simulink model "IEEE9Buses"  (R2024b)
settings: Solver=FixedStepAuto  StartTime=0  StopTime=5  FixedStep=1e-6  RelTol=1e-3
values from neighbouring files (symbols this model uses):
  SG_D_1_D = 0.01056    [SG9_parameters.m]
  SG_D_1_EnableSaturation = 0    [SG9_parameters.m]
  SG_D_1_f0 = 60    [SG9_parameters.m]
  SG_D_1_H = 7.5    [SG9_parameters.m]
  SG_D_1_K_A = 20    [SG9_parameters.m]
  SG_D_1_K_E = 1.000000e+1    (= 10)    [SG9_parameters.m]
  SG_D_1_K_F = 2.363    [SG9_parameters.m]
  SG_D_1_K_s = 5    [SG9_parameters.m]
  SG_D_1_R_a = 0.001088    [SG9_parameters.m]
  SG_D_1_S_A = 1    [SG9_parameters.m]
  SG_D_1_S_B = 0.103    [SG9_parameters.m]
  SG_D_1_S_N = 10.659857    [SG9_parameters.m]
  SG_D_1_SpeedPara = 200    [SG9_parameters.m]
  SG_D_1_T_0 = 0.720173    [SG9_parameters.m]
  SG_D_1_T_1 = 0.3    [SG9_parameters.m]
  SG_D_1_T_2 = 0.05    [SG9_parameters.m]
  SG_D_1_T_3 = 0.02    [SG9_parameters.m]
  SG_D_1_T_4 = 0.005    [SG9_parameters.m]
  SG_D_1_T_A = 0.02    [SG9_parameters.m]
  SG_D_1_T_dd = 8.000000e+0    (= 8)    [SG9_parameters.m]
  SG_D_1_T_ddd = 0.04    [SG9_parameters.m]
  SG_D_1_T_E = 0.314    [SG9_parameters.m]
  SG_D_1_T_F = 0.35    [SG9_parameters.m]
  SG_D_1_T_qd = 0.8    [SG9_parameters.m]
  SG_D_1_T_qdd = 0.02    [SG9_parameters.m]
  SG_D_1_T_speed = 0.1    [SG9_parameters.m]
  SG_D_1_T_w = 0.5    [SG9_parameters.m]
  SG_D_1_V_ref = 1.990276    [SG9_parameters.m]
  SG_D_1_w_ref = 376.991118    [SG9_parameters.m]
  SG_D_1_x_d = 1.9    [SG9_parameters.m]
  SG_D_1_x_dd = 0.302    [SG9_parameters.m]
  SG_D_1_x_ddd = 0.204    [SG9_parameters.m]
  SG_D_1_x_l = 0.05    [SG9_parameters.m]
  SG_D_1_x_q = 1.3    [SG9_parameters.m]
  SG_D_1_x_qd = 0.5    [SG9_parameters.m]
  SG_D_1_x_qdd = 0.3    [SG9_parameters.m]
  SG_D_2_D = 0.01056    [SG9_parameters.m]
  SG_D_2_EnableSaturation = 0    [SG9_parameters.m]
  SG_D_2_f0 = 60    [SG9_parameters.m]
  SG_D_2_H = 7.5    [SG9_parameters.m]
  SG_D_2_K_A = 20    [SG9_parameters.m]
  SG_D_2_K_E = 1.000000e+1    (= 10)    [SG9_parameters.m]
  SG_D_2_K_F = 2.363    [SG9_parameters.m]
  SG_D_2_K_s = 0.5    [SG9_parameters.m]
  SG_D_2_R_a = 0.001088    [SG9_parameters.m]
  SG_D_2_S_A = 1    [SG9_parameters.m]
  SG_D_2_S_B = 0.103    [SG9_parameters.m]
  SG_D_2_S_N = 10.659857    [SG9_parameters.m]
  SG_D_2_SpeedPara = 200    [SG9_parameters.m]
  SG_D_2_T_0 = 1.632913    [SG9_parameters.m]
  SG_D_2_T_1 = 0.2    [SG9_parameters.m]
  SG_D_2_T_2 = 0.05    [SG9_parameters.m]
  SG_D_2_T_3 = 0.02    [SG9_parameters.m]
  SG_D_2_T_4 = 0.005    [SG9_parameters.m]
  SG_D_2_T_A = 0.02    [SG9_parameters.m]
  SG_D_2_T_dd = 8.000000e+0    (= 8)    [SG9_parameters.m]
  SG_D_2_T_ddd = 0.04    [SG9_parameters.m]
  SG_D_2_T_E = 0.314    [SG9_parameters.m]
  SG_D_2_T_F = 0.35    [SG9_parameters.m]
  SG_D_2_T_qd = 0.8    [SG9_parameters.m]
  SG_D_2_T_qdd = 0.02    [SG9_parameters.m]
  SG_D_2_T_speed = 0.1    [SG9_parameters.m]
  SG_D_2_T_w = 0.5    [SG9_parameters.m]
  SG_D_2_V_ref = 2.662631    [SG9_parameters.m]
  SG_D_2_w_ref = 376.991118    [SG9_parameters.m]
  SG_D_2_x_d = 1.9    [SG9_parameters.m]
  SG_D_2_x_dd = 0.302    [SG9_parameters.m]
  SG_D_2_x_ddd = 0.204    [SG9_parameters.m]
  SG_D_2_x_l = 0.05    [SG9_parameters.m]
  SG_D_2_x_q = 1.3    [SG9_parameters.m]
  SG_D_2_x_qd = 0.5    [SG9_parameters.m]
  SG_D_2_x_qdd = 0.3    [SG9_parameters.m]
  SG_D_3_D = 0.01056    [SG9_parameters.m]
  SG_D_3_EnableSaturation = 0    [SG9_parameters.m]
  SG_D_3_f0 = 60    [SG9_parameters.m]
  SG_D_3_H = 7.5    [SG9_parameters.m]
  SG_D_3_K_A = 20    [SG9_parameters.m]
  SG_D_3_K_E = 1.000000e+1    (= 10)    [SG9_parameters.m]
  SG_D_3_K_F = 2.363    [SG9_parameters.m]
  SG_D_3_K_s = 0.5    [SG9_parameters.m]
  SG_D_3_R_a = 0.001088    [SG9_parameters.m]
  SG_D_3_S_A = 1    [SG9_parameters.m]
  SG_D_3_S_B = 0.103    [SG9_parameters.m]
  SG_D_3_S_N = 10.659857    [SG9_parameters.m]
  SG_D_3_SpeedPara = 200    [SG9_parameters.m]
  SG_D_3_T_0 = 0.850788    [SG9_parameters.m]
  SG_D_3_T_1 = 0.2    [SG9_parameters.m]
  SG_D_3_T_2 = 0.05    [SG9_parameters.m]
  SG_D_3_T_3 = 0.02    [SG9_parameters.m]
  SG_D_3_T_4 = 0.005    [SG9_parameters.m]
  SG_D_3_T_A = 0.02    [SG9_parameters.m]
  SG_D_3_T_dd = 8.000000e+0    (= 8)    [SG9_parameters.m]
  SG_D_3_T_ddd = 0.04    [SG9_parameters.m]
  SG_D_3_T_E = 0.314    [SG9_parameters.m]
  SG_D_3_T_F = 0.35    [SG9_parameters.m]
  SG_D_3_T_qd = 0.8    [SG9_parameters.m]
  SG_D_3_T_qdd = 0.02    [SG9_parameters.m]
  SG_D_3_T_speed = 0.1    [SG9_parameters.m]
  SG_D_3_T_w = 0.5    [SG9_parameters.m]
  SG_D_3_V_ref = 1.915682    [SG9_parameters.m]
  SG_D_3_w_ref = 376.991118    [SG9_parameters.m]
  SG_D_3_x_d = 1.9    [SG9_parameters.m]
  SG_D_3_x_dd = 0.302    [SG9_parameters.m]
  SG_D_3_x_ddd = 0.204    [SG9_parameters.m]
  SG_D_3_x_l = 0.05    [SG9_parameters.m]
  SG_D_3_x_q = 1.3    [SG9_parameters.m]
  SG_D_3_x_qd = 0.5    [SG9_parameters.m]
  SG_D_3_x_qdd = 0.3    [SG9_parameters.m]
(part 9 of 9)

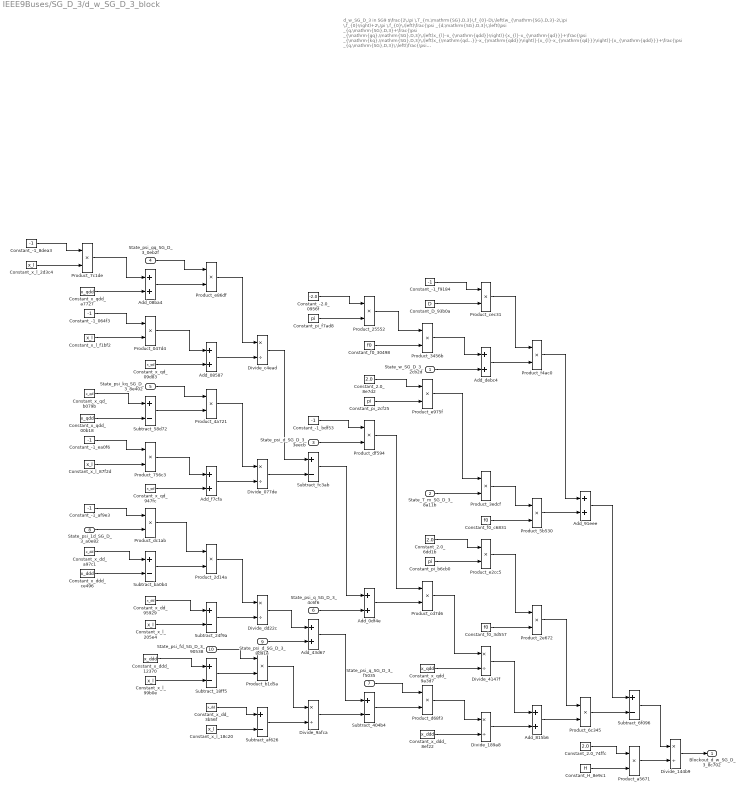
== system IEEE9Buses/SG_D_3/d_w_SG_D_3_block ==
  note: d_w_SG_D_3 in SG9
      | $\frac{2\,\pi \,T_{m,\mathrm{SG},D,3}\,f_{0}-D\,\left(w_{\mathrm{SG},D,3}-2\,\pi \,f_{0}\right)+2\,\pi \,f_{0}\,\left(\frac{\psi _{d,\mathrm{SG},D,3}\,\left(\psi _{q,\mathrm{SG},D,3}+\frac{\psi _{\mathrm{gq},\mathrm{SG},D,3}\,\left(x_{l}-x_{\mathrm{qdd}}\right)}{x_{l}-x_{\mathrm{qd}}}+\frac{\psi _{\mathrm{kq},\mathrm{SG},D,3}\,\left(x_{\mathrm{qd}}-x_{\mathrm{qdd}}\right)}{x_{l}-x_{\mathrm{qd}}}\right)}{x_{\mathrm{qdd}}}+\frac{\psi _{q,\mathrm{SG},D,3}\,\left(\frac{\psi _{\mathrm{1d},\mathrm{SG},D,3}\,\left(x_{\mathrm{dd}}-x_{\mathrm{ddd}}\right)}{x_{\mathrm{dd}}-x_{l}}-\psi _{d,\mathrm{SG},D,3}+\frac{\psi _{\mathrm{fd},\mathrm{SG},D,3}\,\left(x_{\mathrm{ddd}}-x_{l}\right)}{x_{\mathrm{dd}}-x_{l}}\right)}{x_{\mathrm{ddd}}}\right)}{2\,H}$
      | Automatically generated on 2025-09-12 21:33:31 .
  State_w_SG_D_3_2cb2d : Inport
  State_T_m_SG_D_3_8a11b : Inport  Port=2
  State_psi_d_SG_D_3_3eecb : Inport  Port=3
  State_psi_gq_SG_D_3_0eb2f : Inport  Port=4
  State_psi_kq_SG_D_3_8e402 : Inport  Port=5
  State_psi_q_SG_D_3_4c6f6 : Inport  Port=6
  State_psi_q_SG_D_3_f5035 : Inport  Port=7
  State_psi_1d_SG_D_3_a0e82 : Inport  Port=8
  State_psi_d_SG_D_3_8d91e : Inport  Port=9
  State_psi_fd_SG_D_3_90538 : Inport  Port=10
  Add_08587 : Sum
  Add_08ba4 : Sum
  Add_0df4e : Sum
  Add_43d67 : Sum
  Add_815b6 : Sum
  Add_91eee : Sum
  Add_debc4 : Sum
  Add_f7cfa : Sum
  Constant_-1_064f3 : Constant  Value=-1
  Constant_-1_8dea3 : Constant  Value=-1
  Constant_-1_af9e3 : Constant  Value=-1
  Constant_-1_bdf53 : Constant  Value=-1
  Constant_-1_ea0f6 : Constant  Value=-1
  Constant_-1_f9184 : Constant  Value=-1
  Constant_-2.0_0956f : Constant  Value=-2.0
  Constant_2.0_6dd1b : Constant  Value=2.0
  Constant_2.0_74ffc : Constant  Value=2.0
  Constant_2.0_8e7d2 : Constant  Value=2.0
  Constant_D_93b0a : Constant  Value=D
  Constant_H_8e9c1 : Constant  Value=H
  Constant_f0_30498 : Constant  Value=f0
  Constant_f0_3d557 : Constant  Value=f0
  Constant_f0_c6831 : Constant  Value=f0
  Constant_pi_2cf25 : Constant  Value=pi
  Constant_pi_b6cb0 : Constant  Value=pi
  Constant_pi_f7ad8 : Constant  Value=pi
  Constant_x_dd_3b56f : Constant  Value=x_dd
  Constant_x_dd_95929 : Constant  Value=x_dd
  Constant_x_dd_a97c1 : Constant  Value=x_dd
  Constant_x_ddd_12370 : Constant  Value=x_ddd
  Constant_x_ddd_8ef22 : Constant  Value=x_ddd
  Constant_x_ddd_ce496 : Constant  Value=x_ddd
  Constant_x_l_18c20 : Constant  Value=x_l
  Constant_x_l_205e4 : Constant  Value=x_l
  Constant_x_l_2d3c4 : Constant  Value=x_l
  Constant_x_l_87f2d : Constant  Value=x_l
  Constant_x_l_99b0e : Constant  Value=x_l
  Constant_x_l_f1bf2 : Constant  Value=x_l
  Constant_x_qd_09d83 : Constant  Value=x_qd
  Constant_x_qd_947fc : Constant  Value=x_qd
  Constant_x_qd_b079b : Constant  Value=x_qd
  Constant_x_qdd_00b18 : Constant  Value=x_qdd
  Constant_x_qdd_9a3d7 : Constant  Value=x_qdd
  Constant_x_qdd_a7727 : Constant  Value=x_qdd
  Divide_077de : Product  Inputs=*/
  Divide_144b9 : Product  Inputs=*/
  Divide_189a8 : Product  Inputs=*/
  Divide_4147f : Product  Inputs=*/
  Divide_9afca : Product  Inputs=*/
  Divide_c4ead : Product  Inputs=*/
  Divide_dd22c : Product  Inputs=*/
  Product_047d4 : Product
  Product_25552 : Product
  Product_2d14a : Product
  Product_2e672 : Product
  Product_3456b : Product
  Product_3edcf : Product
  Product_4a721 : Product
  Product_5b530 : Product
  Product_6c345 : Product
  Product_756c3 : Product
  Product_7c1de : Product
  Product_a5671 : Product
  Product_b1d5a : Product
  Product_cd7d6 : Product
  Product_cec31 : Product
  Product_d68f3 : Product
  Product_dc1ab : Product
  Product_df594 : Product
  Product_e2cc5 : Product
  Product_e86df : Product
  Product_e975f : Product
  Product_f4ac0 : Product
  Subtract_18ff5 : Sum  Inputs=+-
  Subtract_24f9a : Sum  Inputs=+-
  Subtract_404b4 : Sum  Inputs=+-
  Subtract_58d72 : Sum  Inputs=+-
  Subtract_6f096 : Sum  Inputs=+-
  Subtract_af626 : Sum  Inputs=+-
  Subtract_ba0b4 : Sum  Inputs=+-
  Subtract_fc3ab : Sum  Inputs=+-
  Blockout_d_w_SG_D_3_8c702 : Outport
  wires:
  Constant_x_qd_b079b/1 -> Subtract_58d72/1
  Subtract_ba0b4/1 -> Product_2d14a/2
  Subtract_6f096/1 -> Divide_144b9/1
  Constant_-1_8dea3/1 -> Product_7c1de/1
  Add_08ba4/1 -> Product_e86df/2
  Constant_x_qdd_00b18/1 -> Subtract_58d72/2
  Subtract_18ff5/1 -> Product_b1d5a/2
  Constant_x_l_2d3c4/1 -> Product_7c1de/2
  State_psi_d_SG_D_3_8d91e/1 -> Add_43d67/2
  Add_08587/1 -> Divide_c4ead/2
  Constant_x_dd_95929/1 -> Subtract_24f9a/1
  Constant_x_l_f1bf2/1 -> Product_047d4/2
  Constant_-1_f9184/1 -> Product_cec31/1
  Divide_9afca/1 -> Subtract_404b4/2
  Constant_x_ddd_ce496/1 -> Subtract_ba0b4/2
  Constant_x_qdd_a7727/1 -> Add_08ba4/2
  Constant_pi_2cf25/1 -> Product_e975f/2
  Product_7c1de/1 -> Add_08ba4/1
  Constant_-2.0_0956f/1 -> Product_25552/1
  Constant_-1_064f3/1 -> Product_047d4/1
  Constant_2.0_6dd1b/1 -> Product_e2cc5/1
  Product_25552/1 -> Product_3456b/1
  Constant_-1_ea0f6/1 -> Product_756c3/1
  Subtract_fc3ab/1 -> Add_0df4e/1
  Constant_x_l_87f2d/1 -> Product_756c3/2
  Constant_x_l_99b0e/1 -> Subtract_18ff5/2
  Constant_-1_af9e3/1 -> Product_dc1ab/1
  State_psi_1d_SG_D_3_a0e82/1 -> Product_dc1ab/2
  Constant_x_dd_a97c1/1 -> Subtract_ba0b4/1
  Product_dc1ab/1 -> Product_2d14a/1
  State_psi_gq_SG_D_3_0eb2f/1 -> Product_e86df/1
  Constant_x_qd_09d83/1 -> Add_08587/2
  Product_047d4/1 -> Add_08587/1
  State_psi_kq_SG_D_3_8e402/1 -> Product_4a721/1
  Subtract_58d72/1 -> Product_4a721/2
  Product_e2cc5/1 -> Product_2e672/1
  Product_3456b/1 -> Add_debc4/1
  Product_756c3/1 -> Add_f7cfa/1
  State_psi_q_SG_D_3_f5035/1 -> Product_d68f3/1
  Constant_x_qd_947fc/1 -> Add_f7cfa/2
  Constant_x_l_205e4/1 -> Subtract_24f9a/2
  Constant_x_ddd_12370/1 -> Subtract_18ff5/1
  Constant_x_l_18c20/1 -> Subtract_af626/2
  Product_e86df/1 -> Divide_c4ead/1
  Product_4a721/1 -> Divide_077de/1
  Add_f7cfa/1 -> Divide_077de/2
  Product_2d14a/1 -> Divide_dd22c/1
  Subtract_24f9a/1 -> Divide_dd22c/2
  Constant_2.0_8e7d2/1 -> Product_e975f/1
  State_psi_fd_SG_D_3_90538/1 -> Product_b1d5a/1
  Constant_x_dd_3b56f/1 -> Subtract_af626/1
  Divide_c4ead/1 -> Subtract_fc3ab/1
  Product_b1d5a/1 -> Divide_9afca/1
  Divide_077de/1 -> Subtract_fc3ab/2
  Divide_dd22c/1 -> Add_43d67/1
  Product_6c345/1 -> Subtract_6f096/2
  Subtract_af626/1 -> Divide_9afca/2
  Constant_pi_f7ad8/1 -> Product_25552/2
  Constant_pi_b6cb0/1 -> Product_e2cc5/2
  Constant_-1_bdf53/1 -> Product_df594/1
  State_psi_d_SG_D_3_3eecb/1 -> Product_df594/2
  State_psi_q_SG_D_3_4c6f6/1 -> Add_0df4e/2
  Add_43d67/1 -> Subtract_404b4/1
  Constant_f0_30498/1 -> Product_3456b/2
  Product_df594/1 -> Product_cd7d6/1
  Add_0df4e/1 -> Product_cd7d6/2
  Subtract_404b4/1 -> Product_d68f3/2
  Constant_D_93b0a/1 -> Product_cec31/2
  State_w_SG_D_3_2cb2d/1 -> Add_debc4/2
  Product_e975f/1 -> Product_3edcf/1
  State_T_m_SG_D_3_8a11b/1 -> Product_3edcf/2
  Product_cd7d6/1 -> Divide_4147f/1
  Constant_x_qdd_9a3d7/1 -> Divide_4147f/2
  Product_d68f3/1 -> Divide_189a8/1
  Constant_x_ddd_8ef22/1 -> Divide_189a8/2
  Product_cec31/1 -> Product_f4ac0/1
  Add_debc4/1 -> Product_f4ac0/2
  Product_3edcf/1 -> Product_5b530/1
  Constant_f0_c6831/1 -> Product_5b530/2
  Constant_f0_3d557/1 -> Product_2e672/2
  Divide_4147f/1 -> Add_815b6/1
  Divide_189a8/1 -> Add_815b6/2
  Product_f4ac0/1 -> Add_91eee/1
  Product_5b530/1 -> Add_91eee/2
  Product_2e672/1 -> Product_6c345/1
  Add_815b6/1 -> Product_6c345/2
  Add_91eee/1 -> Subtract_6f096/1
  Constant_2.0_74ffc/1 -> Product_a5671/1
  Constant_H_8e9c1/1 -> Product_a5671/2
  Product_a5671/1 -> Divide_144b9/2
  Divide_144b9/1 -> Blockout_d_w_SG_D_3_8c702/1

== system IEEE9Buses/SG_D_3/i_d_SG_D_3_block ==
  note: i_d_SG_D_3 in SG9
      | $\frac{\sin\left(\theta _{\mathrm{SG},D,3}\right)\,\left(\frac{\psi _{\mathrm{1d},\mathrm{SG},D,3}\,\left(x_{\mathrm{dd}}-x_{\mathrm{ddd}}\right)}{x_{\mathrm{dd}}-x_{l}}-\psi _{d,\mathrm{SG},D,3}+\frac{\psi _{\mathrm{fd},\mathrm{SG},D,3}\,\left(x_{\mathrm{ddd}}-x_{l}\right)}{x_{\mathrm{dd}}-x_{l}}\right)}{x_{\mathrm{ddd}}}-\frac{\cos\left(\theta _{\mathrm{SG},D,3}\right)\,\left(\psi _{q,\mathrm{SG},D,3}+\frac{\psi _{\mathrm{gq},\mathrm{SG},D,3}\,\left(x_{l}-x_{\mathrm{qdd}}\right)}{x_{l}-x_{\mathrm{qd}}}+\frac{\psi _{\mathrm{kq},\mathrm{SG},D,3}\,\left(x_{\mathrm{qd}}-x_{\mathrm{qdd}}\right)}{x_{l}-x_{\mathrm{qd}}}\right)}{x_{\mathrm{qdd}}}$
      | Automatically generated on 2025-09-12 21:33:53 .
  State_psi_gq_SG_D_3_f9205 : Inport
  State_psi_kq_SG_D_3_f6fb5 : Inport  Port=2
  State_psi_q_SG_D_3_097ac : Inport  Port=3
  State_theta_SG_D_3_f2e5f : Inport  Port=4
  State_psi_1d_SG_D_3_3346a : Inport  Port=5
  State_psi_d_SG_D_3_c47d7 : Inport  Port=6
  State_psi_fd_SG_D_3_3705f : Inport  Port=7
  State_theta_SG_D_3_0b124 : Inport  Port=8
  Add_2e819 : Sum
  Add_66e39 : Sum
  Add_78c11 : Sum
  Add_abcc7 : Sum
  Add_c4e16 : Sum
  Constant_-1_12cb5 : Constant  Value=-1
  Constant_-1_21ee1 : Constant  Value=-1
  Constant_-1_82b40 : Constant  Value=-1
  Constant_-1_ad0d8 : Constant  Value=-1
  Constant_-1_b0e43 : Constant  Value=-1
  Constant_x_dd_4f659 : Constant  Value=x_dd
  Constant_x_dd_899e7 : Constant  Value=x_dd
  Constant_x_dd_a714f : Constant  Value=x_dd
  Constant_x_ddd_259a3 : Constant  Value=x_ddd
  Constant_x_ddd_74b9b : Constant  Value=x_ddd
  Constant_x_ddd_a6c9b : Constant  Value=x_ddd
  Constant_x_l_212b9 : Constant  Value=x_l
  Constant_x_l_37c3f : Constant  Value=x_l
  Constant_x_l_510f9 : Constant  Value=x_l
  Constant_x_l_60d37 : Constant  Value=x_l
  Constant_x_l_90ef1 : Constant  Value=x_l
  Constant_x_l_ade82 : Constant  Value=x_l
  Constant_x_qd_06573 : Constant  Value=x_qd
  Constant_x_qd_86486 : Constant  Value=x_qd
  Constant_x_qd_d7580 : Constant  Value=x_qd
  Constant_x_qdd_3a2d2 : Constant  Value=x_qdd
  Constant_x_qdd_a541f : Constant  Value=x_qdd
  Constant_x_qdd_c4b29 : Constant  Value=x_qdd
  Divide_d5013 : Product  Inputs=*/
  Divide_d79b9 : Product  Inputs=*/
  Divide_d802b : Product  Inputs=*/
  Divide_dc0d4 : Product  Inputs=*/
  Divide_e1262 : Product  Inputs=*/
  Divide_f990d : Product  Inputs=*/
  MathFunc_cos_370aa : Trigonometry  Operator=cos
  MathFunc_sin_f020c : Trigonometry
  Product_1432f : Product
  Product_3bfc0 : Product
  Product_457ec : Product
  Product_54605 : Product
  Product_66d72 : Product
  Product_98634 : Product
  Product_9a143 : Product
  Product_b7a28 : Product
  Product_d1de7 : Product
  Product_d2af7 : Product
  Product_d359e : Product
  Subtract_004b3 : Sum  Inputs=+-
  Subtract_01c37 : Sum  Inputs=+-
  Subtract_1435a : Sum  Inputs=+-
  Subtract_4e219 : Sum  Inputs=+-
  Subtract_6b264 : Sum  Inputs=+-
  Subtract_9773a : Sum  Inputs=+-
  Subtract_af2b8 : Sum  Inputs=+-
  Subtract_d3b2c : Sum  Inputs=+-
  Blockout_i_d_SG_D_3_0f9ed : Outport
  wires:
  Constant_x_qd_06573/1 -> Subtract_01c37/1
  Subtract_4e219/1 -> Blockout_i_d_SG_D_3_0f9ed/1
  Constant_-1_ad0d8/1 -> Product_1432f/1
  Constant_x_l_ade82/1 -> Product_457ec/2
  Constant_x_qdd_c4b29/1 -> Add_78c11/2
  Constant_x_qdd_3a2d2/1 -> Subtract_01c37/2
  Constant_x_l_90ef1/1 -> Product_1432f/2
  Divide_d802b/1 -> Subtract_4e219/1
  Product_1432f/1 -> Add_78c11/1
  Constant_x_ddd_74b9b/1 -> Subtract_d3b2c/2
  Constant_-1_b0e43/1 -> Product_457ec/1
  Constant_-1_21ee1/1 -> Product_d2af7/1
  Constant_x_l_212b9/1 -> Product_d2af7/2
  State_psi_1d_SG_D_3_3346a/1 -> Product_98634/2
  State_psi_gq_SG_D_3_f9205/1 -> Product_9a143/1
  Product_98634/1 -> Product_d1de7/1
  Add_78c11/1 -> Product_9a143/2
  Product_457ec/1 -> Add_66e39/1
  Constant_x_qd_d7580/1 -> Add_66e39/2
  State_psi_kq_SG_D_3_f6fb5/1 -> Product_b7a28/1
  Subtract_9773a/1 -> Divide_d5013/2
  Subtract_01c37/1 -> Product_b7a28/2
  Product_d2af7/1 -> Add_2e819/1
  Constant_x_ddd_259a3/1 -> Subtract_004b3/1
  Constant_x_qd_86486/1 -> Add_2e819/2
  Constant_-1_82b40/1 -> Product_98634/1
  Constant_x_dd_4f659/1 -> Subtract_d3b2c/1
  Product_9a143/1 -> Divide_f990d/1
  Add_66e39/1 -> Divide_f990d/2
  Product_b7a28/1 -> Divide_dc0d4/1
  Add_2e819/1 -> Divide_dc0d4/2
  Divide_d5013/1 -> Subtract_af2b8/2
  Subtract_d3b2c/1 -> Product_d1de7/2
  State_theta_SG_D_3_f2e5f/1 -> MathFunc_cos_370aa/1
  Constant_x_dd_899e7/1 -> Subtract_6b264/1
  Product_3bfc0/1 -> Product_54605/1
  Constant_x_l_510f9/1 -> Subtract_6b264/2
  Add_c4e16/1 -> Subtract_af2b8/1
  Constant_x_l_37c3f/1 -> Subtract_004b3/2
  State_theta_SG_D_3_0b124/1 -> MathFunc_sin_f020c/1
  Divide_f990d/1 -> Subtract_1435a/1
  Add_abcc7/1 -> Product_3bfc0/2
  Divide_dc0d4/1 -> Subtract_1435a/2
  Product_d1de7/1 -> Divide_e1262/1
  Subtract_6b264/1 -> Divide_e1262/2
  State_psi_fd_SG_D_3_3705f/1 -> Product_d359e/1
  Divide_d79b9/1 -> Subtract_4e219/2
  Subtract_004b3/1 -> Product_d359e/2
  Constant_x_dd_a714f/1 -> Subtract_9773a/1
  Subtract_1435a/1 -> Add_abcc7/1
  Constant_x_l_60d37/1 -> Subtract_9773a/2
  Constant_-1_12cb5/1 -> Product_3bfc0/1
  State_psi_q_SG_D_3_097ac/1 -> Add_abcc7/2
  Divide_e1262/1 -> Add_c4e16/1
  State_psi_d_SG_D_3_c47d7/1 -> Add_c4e16/2
  Product_d359e/1 -> Divide_d5013/1
  MathFunc_cos_370aa/1 -> Product_54605/2
  MathFunc_sin_f020c/1 -> Product_66d72/2
  Subtract_af2b8/1 -> Product_66d72/1
  Product_54605/1 -> Divide_d802b/1
  Constant_x_qdd_a541f/1 -> Divide_d802b/2
  Product_66d72/1 -> Divide_d79b9/1
  Constant_x_ddd_a6c9b/1 -> Divide_d79b9/2

== system IEEE9Buses/SG_D_3/i_q_SG_D_3_block ==
  note: i_q_SG_D_3 in SG9
      | $-\frac{\sin\left(\theta _{\mathrm{SG},D,3}\right)\,\left(\psi _{q,\mathrm{SG},D,3}+\frac{\psi _{\mathrm{gq},\mathrm{SG},D,3}\,\left(x_{l}-x_{\mathrm{qdd}}\right)}{x_{l}-x_{\mathrm{qd}}}+\frac{\psi _{\mathrm{kq},\mathrm{SG},D,3}\,\left(x_{\mathrm{qd}}-x_{\mathrm{qdd}}\right)}{x_{l}-x_{\mathrm{qd}}}\right)}{x_{\mathrm{qdd}}}-\frac{\cos\left(\theta _{\mathrm{SG},D,3}\right)\,\left(\frac{\psi _{\mathrm{1d},\mathrm{SG},D,3}\,\left(x_{\mathrm{dd}}-x_{\mathrm{ddd}}\right)}{x_{\mathrm{dd}}-x_{l}}-\psi _{d,\mathrm{SG},D,3}+\frac{\psi _{\mathrm{fd},\mathrm{SG},D,3}\,\left(x_{\mathrm{ddd}}-x_{l}\right)}{x_{\mathrm{dd}}-x_{l}}\right)}{x_{\mathrm{ddd}}}$
      | Automatically generated on 2025-09-12 21:33:57 .
  State_psi_gq_SG_D_3_7b6eb : Inport
  State_psi_kq_SG_D_3_c33f6 : Inport  Port=2
  State_psi_q_SG_D_3_85401 : Inport  Port=3
  State_theta_SG_D_3_ac3c7 : Inport  Port=4
  State_psi_1d_SG_D_3_c21a4 : Inport  Port=5
  State_psi_d_SG_D_3_d5142 : Inport  Port=6
  State_psi_fd_SG_D_3_e8d39 : Inport  Port=7
  State_theta_SG_D_3_89a28 : Inport  Port=8
  Add_002fd : Sum
  Add_31654 : Sum
  Add_5954b : Sum
  Add_ae96f : Sum
  Add_b7055 : Sum
  Add_f7e99 : Sum
  Constant_-1_17a1f : Constant  Value=-1
  Constant_-1_4de8a : Constant  Value=-1
  Constant_-1_8ccdc : Constant  Value=-1
  Constant_-1_90ffb : Constant  Value=-1
  Constant_-1_ab62d : Constant  Value=-1
  Constant_x_dd_1ab0a : Constant  Value=x_dd
  Constant_x_dd_1ef45 : Constant  Value=x_dd
  Constant_x_dd_a2115 : Constant  Value=x_dd
  Constant_x_ddd_12962 : Constant  Value=x_ddd
  Constant_x_ddd_9466a : Constant  Value=x_ddd
  Constant_x_ddd_dde30 : Constant  Value=x_ddd
  Constant_x_l_0aa3f : Constant  Value=x_l
  Constant_x_l_0c368 : Constant  Value=x_l
  Constant_x_l_16c34 : Constant  Value=x_l
  Constant_x_l_394b8 : Constant  Value=x_l
  Constant_x_l_90520 : Constant  Value=x_l
  Constant_x_l_e5c76 : Constant  Value=x_l
  Constant_x_qd_2e3b5 : Constant  Value=x_qd
  Constant_x_qd_30ae7 : Constant  Value=x_qd
  Constant_x_qd_92aec : Constant  Value=x_qd
  Constant_x_qdd_2fd0f : Constant  Value=x_qdd
  Constant_x_qdd_dc6c6 : Constant  Value=x_qdd
  Constant_x_qdd_ec1a5 : Constant  Value=x_qdd
  Divide_2aa35 : Product  Inputs=*/
  Divide_3aef0 : Product  Inputs=*/
  Divide_43ac2 : Product  Inputs=*/
  Divide_4c791 : Product  Inputs=*/
  Divide_65aaa : Product  Inputs=*/
  Divide_9aaca : Product  Inputs=*/
  MathFunc_cos_a46a9 : Trigonometry  Operator=cos
  MathFunc_sin_be254 : Trigonometry
  Product_09edf : Product
  Product_1f604 : Product
  Product_5a4ef : Product
  Product_69c5d : Product
  Product_6a0f2 : Product
  Product_74a43 : Product
  Product_99a48 : Product
  Product_b4662 : Product
  Product_e69c9 : Product
  Product_eb5b4 : Product
  Product_f8603 : Product
  Subtract_42e16 : Sum  Inputs=+-
  Subtract_877dd : Sum  Inputs=+-
  Subtract_95f44 : Sum  Inputs=+-
  Subtract_b4637 : Sum  Inputs=+-
  Subtract_d1505 : Sum  Inputs=+-
  Subtract_e6809 : Sum  Inputs=+-
  Subtract_ee4ea : Sum  Inputs=+-
  Blockout_i_q_SG_D_3_01fe5 : Outport
  wires:
  Constant_x_qdd_ec1a5/1 -> Divide_3aef0/2
  Constant_x_dd_1ef45/1 -> Subtract_95f44/1
  Constant_-1_90ffb/1 -> Product_b4662/1
  Constant_-1_17a1f/1 -> Product_eb5b4/1
  Constant_x_l_0c368/1 -> Product_eb5b4/2
  Subtract_d1505/1 -> Product_74a43/1
  Constant_x_qdd_dc6c6/1 -> Subtract_e6809/2
  Constant_x_qdd_2fd0f/1 -> Add_ae96f/2
  Product_eb5b4/1 -> Add_ae96f/1
  Constant_x_l_0aa3f/1 -> Subtract_95f44/2
  Add_5954b/1 -> Divide_4c791/2
  Constant_x_l_e5c76/1 -> Product_b4662/2
  Constant_x_ddd_12962/1 -> Subtract_b4637/1
  Constant_x_qd_30ae7/1 -> Subtract_e6809/1
  Constant_-1_ab62d/1 -> Product_f8603/1
  Product_1f604/1 -> Product_6a0f2/1
  Constant_x_l_90520/1 -> Product_f8603/2
  Product_6a0f2/1 -> Divide_43ac2/1
  State_psi_gq_SG_D_3_7b6eb/1 -> Product_99a48/1
  Add_ae96f/1 -> Product_99a48/2
  Subtract_95f44/1 -> Divide_43ac2/2
  Product_b4662/1 -> Add_5954b/1
  Divide_2aa35/1 -> Add_31654/2
  Constant_x_qd_92aec/1 -> Add_5954b/2
  State_psi_fd_SG_D_3_e8d39/1 -> Product_69c5d/1
  State_psi_kq_SG_D_3_c33f6/1 -> Product_09edf/1
  Subtract_b4637/1 -> Product_69c5d/2
  Subtract_e6809/1 -> Product_09edf/2
  Product_f8603/1 -> Add_b7055/1
  Constant_x_qd_2e3b5/1 -> Add_b7055/2
  Constant_x_l_16c34/1 -> Subtract_b4637/2
  Constant_-1_8ccdc/1 -> Product_1f604/1
  State_psi_1d_SG_D_3_c21a4/1 -> Product_1f604/2
  Constant_x_dd_1ab0a/1 -> Subtract_877dd/1
  Constant_-1_4de8a/1 -> Product_5a4ef/1
  Constant_x_ddd_dde30/1 -> Subtract_877dd/2
  Add_f7e99/1 -> Product_5a4ef/2
  Product_99a48/1 -> Divide_4c791/1
  Product_69c5d/1 -> Divide_9aaca/1
  Product_09edf/1 -> Divide_65aaa/1
  Subtract_ee4ea/1 -> Divide_9aaca/2
  Add_b7055/1 -> Divide_65aaa/2
  Constant_x_ddd_9466a/1 -> Divide_2aa35/2
  Subtract_877dd/1 -> Product_6a0f2/2
  Divide_4c791/1 -> Subtract_42e16/1
  Divide_9aaca/1 -> Subtract_d1505/2
  Divide_65aaa/1 -> Subtract_42e16/2
  Constant_x_dd_a2115/1 -> Subtract_ee4ea/1
  Constant_x_l_394b8/1 -> Subtract_ee4ea/2
  Subtract_42e16/1 -> Add_f7e99/1
  State_psi_q_SG_D_3_85401/1 -> Add_f7e99/2
  Divide_43ac2/1 -> Add_002fd/1
  MathFunc_sin_be254/1 -> Product_e69c9/2
  Product_5a4ef/1 -> Product_e69c9/1
  State_psi_d_SG_D_3_d5142/1 -> Add_002fd/2
  State_theta_SG_D_3_ac3c7/1 -> MathFunc_sin_be254/1
  Add_002fd/1 -> Subtract_d1505/1
  State_theta_SG_D_3_89a28/1 -> MathFunc_cos_a46a9/1
  MathFunc_cos_a46a9/1 -> Product_74a43/2
  Divide_3aef0/1 -> Add_31654/1
  Product_e69c9/1 -> Divide_3aef0/1
  Product_74a43/1 -> Divide_2aa35/1
  Add_31654/1 -> Blockout_i_q_SG_D_3_01fe5/1

== system IEEE9Buses/SG_D_3/theta_SG_D_3_out_block ==
  note: theta_SG_D_3_out in SG9
      | $\theta _{\mathrm{SG},D,3}$
      | Automatically generated on 2025-09-12 21:34:02 .
  State_theta_SG_D_3_cae6d : Inport
  Blockout_theta_SG_D_3_out_1963e : Outport
  wires:
  State_theta_SG_D_3_cae6d/1 -> Blockout_theta_SG_D_3_out_1963e/1

== system IEEE9Buses/SG_D_3/w_SG_D_3_out_block ==
  note: w_SG_D_3_out in SG9
      | $w_{\mathrm{SG},D,3}$
      | Automatically generated on 2025-09-12 21:34:01 .
  State_w_SG_D_3_bbd42 : Inport
  Blockout_w_SG_D_3_out_93636 : Outport
  wires:
  State_w_SG_D_3_bbd42/1 -> Blockout_w_SG_D_3_out_93636/1
